simulink model "PE_pro"  (R2021b)
settings: Solver=VariableStepAuto  StartTime=0.0  StopTime=T  RelTol=1e-3
values from neighbouring files (symbols this model uses):
  F = (angle/step_angle)*sample_time    (= 0.0555555555556)    [inputs.m]
  in1 = [1 0 0 1]    [inputs.m]
  in2 = ~in1    [inputs.m]
  in3 = [ 1 1 0 0]    [inputs.m]
  in4 = ~in3    [inputs.m]
  velocity = 30    [inputs.m]
libraries: simulink x8, spsMosfetLib x8, spsDCVoltageSourceLib x2, spsGroundLib x2, spsStepperMotorLib x1, spspowerguiLib x1
settings Model: Creator=ASUS  LastModifiedBy=ASUS

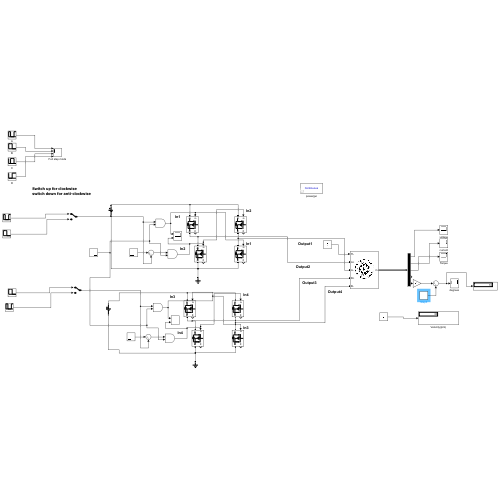
[thumbnail: Simulink's stored preview of the top-level diagram]
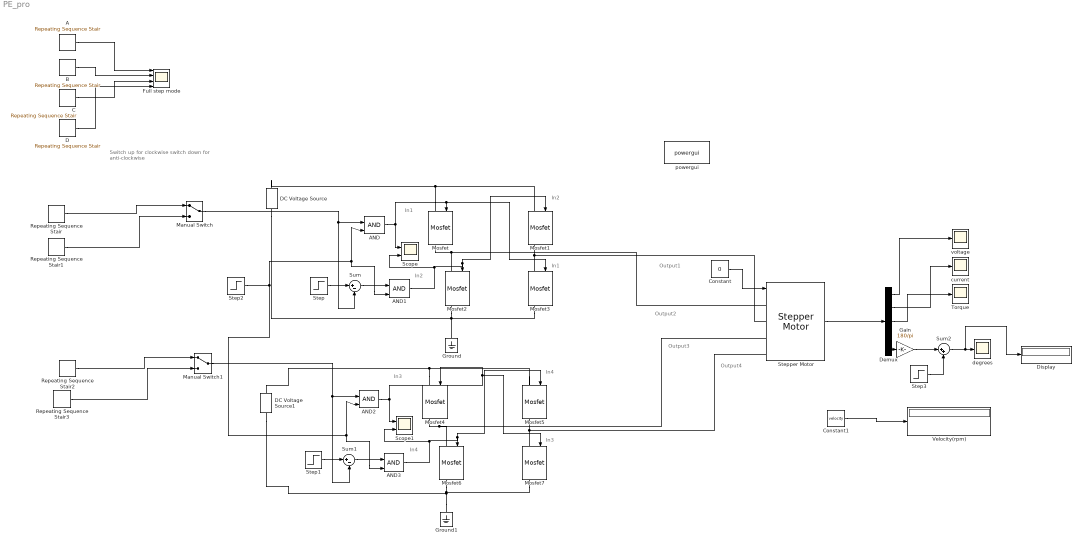
== system PE_pro ==
  note: Switch up for clockwise
      | switch down for anti-clockwise
  note: Output1
  note: In1
  note: In2
  note: In1
  note: In2
  note: In3
  note: In4
  note: Output2
  note: Output3
  note: Output4
  note: In4
  note: In3
  A : simulink/Sources/Repeating Sequence Stair  OutValues=in1.'  tsamp=S  OutMin=[]  OutMax=[]  OutDataTypeStr=double  OutputDataTypeScalingMode=double  OutDataType=fixdt(0,8)  ConRadixGroup=Best Precision: Vector-wise  OutScaling=2^-12
  AND{,1..3} (4 alike) : Logic  IconShape=distinctive  AllPortsSameDT=off  OutDataTypeStr=boolean
  B : simulink/Sources/Repeating Sequence Stair  OutValues=in3.'  tsamp=S  OutMin=[]  OutMax=[]  OutDataTypeStr=double  OutputDataTypeScalingMode=double  OutDataType=fixdt(0,8)  ConRadixGroup=Best Precision: Vector-wise  OutScaling=2^-12
  C : simulink/Sources/Repeating Sequence Stair  OutValues=in2.'  tsamp=S  OutMin=[]  OutMax=[]  OutDataTypeStr=double  OutputDataTypeScalingMode=double  OutDataType=fixdt(0,8)  ConRadixGroup=Best Precision: Vector-wise  OutScaling=2^-12
  Constant : Constant  Value=0
  Constant1 : Constant  Value=velocity
  D : simulink/Sources/Repeating Sequence Stair  OutValues=in4.'  tsamp=S  OutMin=[]  OutMax=[]  OutDataTypeStr=double  OutputDataTypeScalingMode=double  OutDataType=fixdt(0,8)  ConRadixGroup=Best Precision: Vector-wise  OutScaling=2^-12
  DC Voltage Source : spsDCVoltageSourceLib/DC Voltage Source  Amplitude=100  Measurements=None
  DC Voltage Source1 : spsDCVoltageSourceLib/DC Voltage Source  Amplitude=100  Measurements=None
  Demux : Demux  Outputs=5
  Display : Display
  Full step mode : Scope  NumInputPorts=4
  Gain : Gain  Gain=180/pi
  Ground : spsGroundLib/Ground  LConnTagsString=a
  Ground1 : spsGroundLib/Ground  LConnTagsString=a
  Manual Switch : ManualSwitch
  Manual Switch1 : ManualSwitch
  Mosfet{,1..7} (8 alike) : spsMosfetLib/Mosfet  Ron=0.1  Lon=0  Rd=0.01  Vfd=0  IC=0  Rs=1e5  Cs=inf  Measurements=on
  Repeating Sequence Stair : simulink/Sources/Repeating Sequence Stair  OutValues=in1.'  tsamp=S  OutMin=[]  OutMax=[]  OutDataTypeStr=double  OutputDataTypeScalingMode=double  OutDataType=fixdt(0,8)  ConRadixGroup=Best Precision: Vector-wise  OutScaling=2^-12
  Repeating Sequence Stair1 : simulink/Sources/Repeating Sequence Stair  OutValues=in3.'  tsamp=S  OutMin=[]  OutMax=[]  OutDataTypeStr=double  OutputDataTypeScalingMode=double  OutDataType=fixdt(0,8)  ConRadixGroup=Best Precision: Vector-wise  OutScaling=2^-12
  Repeating Sequence Stair2 : simulink/Sources/Repeating Sequence Stair  OutValues=in3.'  tsamp=S  OutMin=[]  OutMax=[]  OutDataTypeStr=double  OutputDataTypeScalingMode=double  OutDataType=fixdt(0,8)  ConRadixGroup=Best Precision: Vector-wise  OutScaling=2^-12
  Repeating Sequence Stair3 : simulink/Sources/Repeating Sequence Stair  OutValues=in1.'  tsamp=S  OutMin=[]  OutMax=[]  OutDataTypeStr=double  OutputDataTypeScalingMode=double  OutDataType=fixdt(0,8)  ConRadixGroup=Best Precision: Vector-wise  OutScaling=2^-12
  Scope : Scope  NumInputPorts=2
  Scope1 : Scope  NumInputPorts=2
  Step : Step  Time=0  SampleTime=0
  Step1 : Step  Time=0  SampleTime=0
  Step2 : Step  Time=F  Before=1  After=0  SampleTime=0
  Step3 : Step  Time=0  SampleTime=0
  Stepper Motor : spsStepperMotorLib/Stepper Motor  MotorType=Permanent-magnet / Hybrid  NumberOfPhases_1=2  NumberOfPhases_2=3  PresetModel_1=<empty>  PresetModel_2=<empty>  L=10e-3  Lmax=10e-3  Lmin=2e-3  R=1.2  Step_angle=step_angle  Psim=0.04  Tdm=0.02  J=1e-4/5  B=1e-3  w0=0  pos0=0  TsPowergui=0  TsBlock=-1
      settings: SourceProductBaseCode=PS
  Sum : Sum  Inputs=|+-
  Sum1 : Sum  Inputs=|+-
  Sum2 : Sum  Inputs=|++
  Torque : Scope
  Velocity(rpm) : Display
  current : Scope
  degrees : Scope
  powergui : spspowerguiLib/powergui  Priority=1  SimulationMode=Continuous  SampleTime=50e-6  frequency=60  Iterations=50  frequencyindice=0  Pbase=100e6  ErrMax=1e-4  UnitsV=kV  UnitsW=MW  buscounter=0  FunctionMessages=off  echomessages=off  EnableUseOfTLC=off  CurrentSourceSwitches=off  DisableSnubberDevices=off  DisableRonSwitches=off  DisableVfSwitches=off  DisplayEquations=off  AutomaticDiscreteSolvers=off  SolverType=Tustin/Backward Euler (TBE)  Interpol=off  ExternalGateDelay=off  methode=off  Ts=100  x0status=blocks  SPID=on  SwTol=0  HookPort=off  NonlinearTolerance=1e-4  nMaxIteration=100  ContinueOnMaxIteration=off  RestoreLinks=warning  ResistiveCurrentMeasurement=off  Frange=[0:2:500]  Ylog=off  Xlog=on  ShowGrid=off  save=off  variable=ZData  structure=0  ZoomFFT=off  StartTime=0.0  cycles=1  DisplayStyle=1  fundamental=60  FreqAxis=off  MaxFrequency=1000  frequencyindicesteady=1  RmsSteady=1  display=off
  voltage : Scope
  wires:
  Step/1 -> Sum/1
  Constant/1 -> Stepper Motor/1
  Manual Switch/1 -> AND/1, Sum/2
  Sum/1 -> AND1/1
  AND1/1 -> Mosfet1/1, Mosfet2/1, Scope/2
  AND/1 -> Scope/1, Mosfet3/1, Mosfet/1
  AND3/1 -> Mosfet5/1, Mosfet6/1, Scope1/2
  AND2/1 -> Scope1/1, Mosfet7/1, Mosfet4/1
  Sum1/1 -> AND3/1
  Manual Switch1/1 -> AND2/1, Sum1/2
  Step2/1 -> AND3/2, AND2/2, AND1/2, AND/2
  Step1/1 -> Sum1/1
  Stepper Motor/1 -> Demux/1
  Demux/5 -> Gain/1
  Demux/3 -> Torque/1
  Demux/2 -> current/1
  Demux/1 -> voltage/1
  Repeating Sequence Stair1/1 -> Manual Switch/2
  Repeating Sequence Stair/1 -> Manual Switch/1
  Repeating Sequence Stair3/1 -> Manual Switch1/2
  Repeating Sequence Stair2/1 -> Manual Switch1/1
  A/1 -> Full step mode/1
  B/1 -> Full step mode/2
  C/1 -> Full step mode/3
  D/1 -> Full step mode/4
  Constant1/1 -> Velocity(rpm)/1
  Gain/1 -> Sum2/1
  Step3/1 -> Sum2/2
  Sum2/1 -> Display/1, degrees/1
  connections:
  Mosfet/RConn1 -- Stepper Motor/LConn1 -- Mosfet2/LConn1
  Mosfet2/RConn1 -- Mosfet3/RConn1 -- DC Voltage Source/LConn1 -- Ground/LConn1
  Mosfet1/RConn1 -- Stepper Motor/LConn2 -- Mosfet3/LConn1
  Mosfet/LConn1 -- DC Voltage Source/RConn1 -- Mosfet1/LConn1
  Ground1/LConn1 -- DC Voltage Source1/LConn1 -- Mosfet7/RConn1 -- Mosfet6/RConn1
  Mosfet5/RConn1 -- Stepper Motor/LConn4 -- Mosfet7/LConn1
  Mosfet4/LConn1 -- DC Voltage Source1/RConn1 -- Mosfet5/LConn1
  Mosfet4/RConn1 -- Stepper Motor/LConn3 -- Mosfet6/LConn1
